simulink model "degree"  (R2014a)
settings: Solver=FixedStepDiscrete  StartTime=0.0  StopTime=60  FixedStep=0.001  RelTol=1e-3
libraries: dspswit3 x3, xpcnilib x2, slrtlib x2, simulink x1
settings Model: SimulationMode=external  BufferReuse=off  Creator=Lab322  LastModifiedBy=Lab322
settings SolverCC: EnableConcurrentExecution=on
settings OptimizationCC: BlockReduction=off  OptimizeBlockIOStorage=off  BufferReuse=off  GlobalBufferReuse=off  ExpressionFolding=off  LocalBlockOutputs=off
settings HardwareCC: ProdIntDivRoundTo=Zero  ProdEndianess=LittleEndian  ProdHWDeviceType=Generic->32-bit x86 compatible
settings RTWCC: SystemTargetFile=slrt.tlc  TemplateMakefile=slrt_default_tmf  Description=Simulink Real-Time  ProcessScript=slrt_make_rtw_hook  RTWCompilerOptimization=On
settings SimulinkRealTimeCC: GeneratePreprocessorConditionals=Disable all  EnableShiftOperators=on

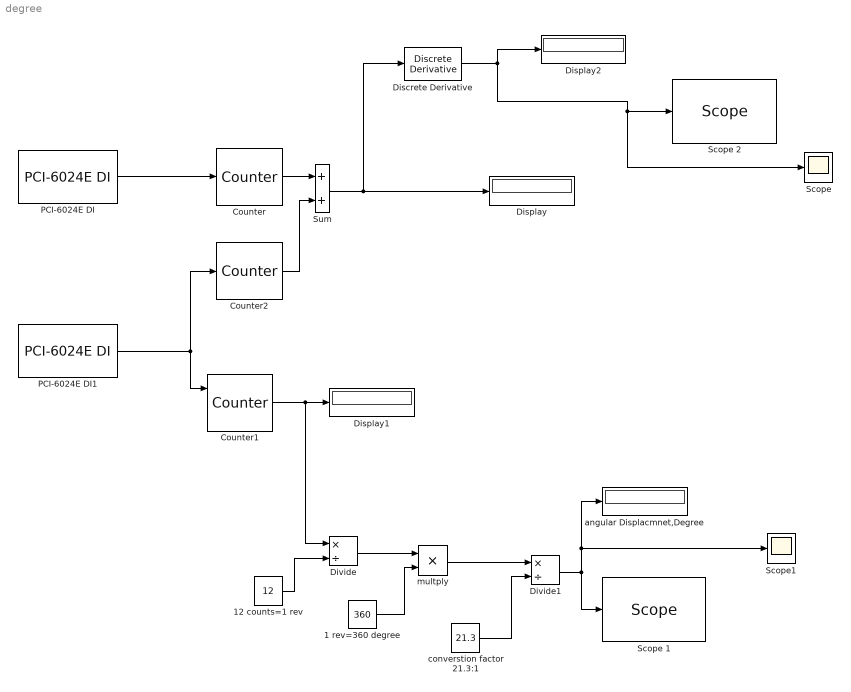
== system degree ==
  1 rev=360 degree : Constant  Value=360
  12 counts=1 rev : Constant  Value=12
  Counter : dspswit3/Counter  Direction=Up  CountEvent=Rising edge  CounterSize=32 bits  MaxCount=255  InitialCount=0  Output=Count  HitValue=32  ResetInput=off  SamplesPerFrame=1  Ts=1  CntDtype=double  HitDtype=Logical
  Counter1 : dspswit3/Counter  Direction=Up  CountEvent=Rising edge  CounterSize=32 bits  MaxCount=255  InitialCount=0  Output=Count  HitValue=32  ResetInput=on  SamplesPerFrame=1  Ts=1  CntDtype=double  HitDtype=Logical
  Counter2 : dspswit3/Counter  Direction=Up  CountEvent=Rising edge  CounterSize=32 bits  MaxCount=255  InitialCount=0  Output=Count  HitValue=32  ResetInput=off  SamplesPerFrame=1  Ts=1  CntDtype=double  HitDtype=Logical
  Discrete Derivative : simulink/Discrete/Discrete Derivative  gainval=1.0  ICPrevScaledInput=0.0  InputProcessing=Inherited  OutMin=[]  OutMax=[]  OutDataType=fixdt(1, 16)  OutScaling=2^-10  DoSatur=off
  Display : Display
  Display1 : Display
  Display2 : Display
  Divide : Product  Inputs=*/
  Divide1 : Product  Inputs=*/
  PCI-6024E DI : xpcnilib/Digital Input/E Series/PCI-6024E DI  channel=[7]  sampletime=0.001  slot=-1
  PCI-6024E DI1 : xpcnilib/Digital Input/E Series/PCI-6024E DI  channel=[8]  sampletime=0.001  slot=-1
  Scope : Scope
  Scope 1 : slrtlib/Displays and Logging/Scope   scopeno=2  scopetype=Target  autostart=on  viewmode=Graphical redraw  formatstr='%15.6f'  grid=on  ylimits=[0,0]  nosamples=600  noprepostsamples=0  interleave=1  triggermode=FreeRun  triggersignal=1  trigsignalfromport=off  triggerlevel=0.0  triggerslope=Either  triggerscope=1  triggersample=0  filename=data.dat  mode=Lazy  writesize=512  autorestart=off  dynamicfilemode=off  maxwritefilesize=512*1024^2
  Scope 2 : slrtlib/Displays and Logging/Scope   scopeno=3  scopetype=Target  autostart=on  viewmode=Graphical redraw  formatstr='%15.6f'  grid=on  ylimits=[0,0]  nosamples=600  noprepostsamples=0  interleave=1  triggermode=FreeRun  triggersignal=1  trigsignalfromport=off  triggerlevel=0.0  triggerslope=Either  triggerscope=1  triggersample=0  filename=data.dat  mode=Lazy  writesize=512  autorestart=off  dynamicfilemode=off  maxwritefilesize=512*1024^2
  Scope1 : Scope
  Sum : Sum
  angular Displacmnet,Degree : Display
  converstion factor 21.3:1 : Constant  Value=21.3
  multply : Product  Inputs=**
  wires:
  PCI-6024E DI1/1 -> Counter1/1, Counter2/1
  PCI-6024E DI/1 -> Counter/1
  Counter1/1 -> Divide/1, Display1/1
  Discrete Derivative/1 -> Display2/1, Scope/1, Scope 2/1
  12 counts=1 rev/1 -> Divide/2
  converstion factor 21.3:1/1 -> Divide1/2
  multply/1 -> Divide1/1
  Divide/1 -> multply/1
  1 rev=360 degree/1 -> multply/2
  Divide1/1 -> Scope1/1, angular Displacmnet,Degree/1, Scope 1/1
  Counter/1 -> Sum/1
  Sum/1 -> Discrete Derivative/1, Display/1
  Counter2/1 -> Sum/2
